simulink model "overtake_QCar"  (R2021a)
settings: Solver=ode1  StartTime=0.0  StopTime=11  FixedStep=1/30  RelTol=1e-3  EnableMultiTasking=on
values from neighbouring files (symbols this model uses):
  animation_update_interval = C*h_fixed    [setup_TP.m]
  enable_CG_trace = 1    [setup_TP.m]
  enable_rearAxle_trace = 1    [setup_TP.m]
  plotAxisLimitMode = 0    [setup_TP.m]
  plotAxisLimits = [-3 4 -3 5]    [setup_TP.m]
  save_anim_frames = 0    [setup_TP.m]
  vehicle_length = 0.256    [setup_TP.m]
  vehicle_width = 0.170    (= 0.17)    [setup_TP.m]
  x0 = [2 6 pi/2]    [setup_TP.m]
undefined symbols (not defined in the file or in its folder): datetime, HIL
libraries: quarc_library x5, simulink x2
settings Model: SimulationMode=external  ExtModeTrigDuration=10000  Creator=Quanser  LastModifiedBy=User
settings SolverCC: AlgebraicLoopSolver=TrustRegion  PositivePriorityOrder=on
settings DataIOCC: ReturnWorkspaceOutputs=off
settings DebuggingCC: PregeneratedLibrarySubsystemCodeDiagnostic=none  SFMachineParentedDataDiag=warning  ArithmeticOperatorsInVariantConditions=warning
settings HardwareCC: ProdBitPerLong=64  ProdLargestAtomicInteger=LongLong  ProdLargestAtomicFloat=Double  ProdLongLongMode=on  ProdHWDeviceType=ARM Compatible->ARM 64-bit (LP64)
settings SFSimCC: CustomCodeUndefinedFunction=UseInterfaceOnly
settings RTWCC: Description=QUARC Linux Nvidia Target (QCar) Using Toolchain  SystemTargetFile=quarc_linux_nvidia.tlc  TemplateMakefile=quarc_default_tmf  Toolchain=QUARC linux_nvidia | gmake (64-bit Windows)  BuildConfiguration=Faster Runs
settings STFCustomTargetCC: TargetLangStandard=C99 (ISO)  ConcurrentExecutionCompliant=on  SystemTargetFile=quarc_linux_nvidia.tlc
settings GRTTargetCC: ParMdlRefBuildCompliant=off  CompOptLevelCompliant=off  CombineOutputUpdateFcns=off  MatFileLogging=off  CPPClassGenCompliant=off  GRTInterface=on  ExtMode=on  ExtModeMexFile=quarc_comm  ExtModeMexArgs='-w -d /tmp -uri %u','tcpip://192.168.2.12:17001'

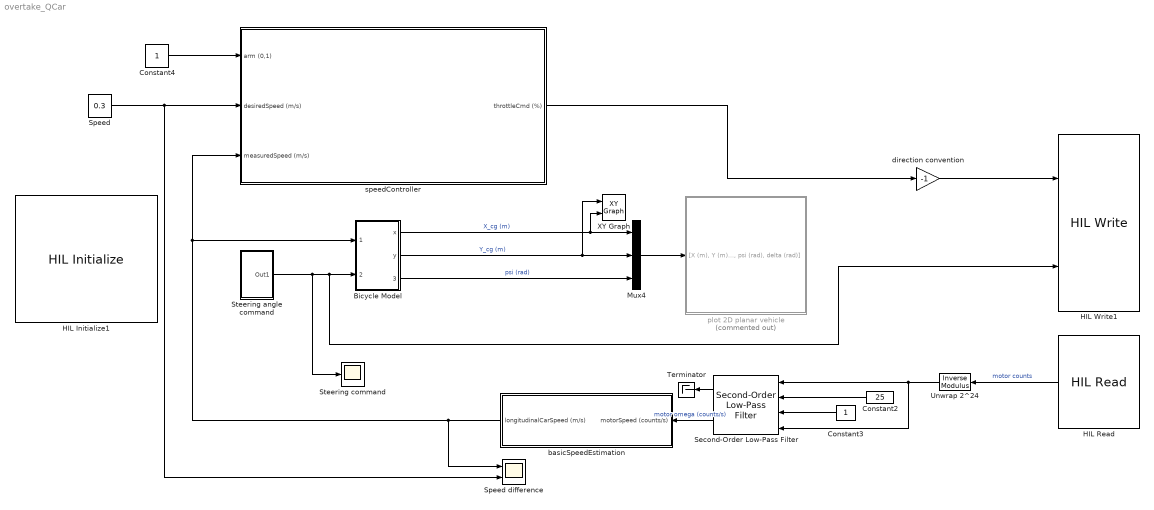
== system overtake_QCar ==
  Bicycle Model : Subsystem
  Constant2 : Constant  Value=25
  Constant3 : Constant
  Constant4 : Constant  VectorParams1D=off
  HIL Initialize1 : quarc_library/Data Acquisition/Generic/Configuration/HIL Initialize  object_name=HIL-1  board_type=qcar  board_number=0  board_options=gyro_fs=125;gyro_rate=47;accel_fs=2;accel_rate=62.5;mag_rate=20;mag_xy=47;mag_z=83;enc1_dir=0;enc2_dir=0;enc3_dir=0;enc4_dir=0;pwm1_dshot=0;pwm2_dshot=0;pwm3_dshot=0;pwm4_dshot=0;pwm5_dshot=0;pwm6_dshot=0;pwm7_dshot=0;steer_bias=0.05;motor_limit=0.3;  exclusive=off  active=on  hardware_clocks=[]  clock_modes=[]  initial_clock_frequencies=[]  set_clock_params_at_start=off  set_clock_params_at_switch_in=off  set_clock_frequencies_at_start=off  set_clock_frequencies_at_switch_in=off  analog_input_channels=[0:6]  analog_input_configurations=[]  analog_input_maximums=[3.3]  analog_input_minimums=[0]  set_analog_input_params_at_start=off  set_analog_input_params_at_switch_in=off  analog_output_channels=[]  analog_output_maximums=[]  analog_output_minimums=[]  initial_analog_outputs=[]  final_analog_outputs=[]  watchdog_analog_outputs=[]  set_analog_output_params_at_start=off  set_analog_output_params_at_switch_in=off  set_analog_outputs_at_start=off  set_analog_outputs_at_switch_in=off  set_analog_outputs_at_terminate=off  set_analog_outputs_at_switch_out=off  set_analog_outputs_on_watchdog=off  digital_input_channels=[24:43]  digital_output_channels=[40]  digital_output_configuration=[]  initial_digital_outputs=[0]  final_digital_outputs=[1]  watchdog_digital_outputs=[]  set_digital_output_params_at_start=off  set_digital_output_params_at_switch_in=off  set_digital_outputs_at_start=on  set_digital_outputs_at_switch_in=off  set_digital_outputs_at_terminate=on  set_digital_outputs_at_switch_out=off  set_digital_outputs_on_watchdog=off  encoder_channels=[0:4]  quadrature=[4 4]  encoder_filter_frequency=100e6/1  initial_encoder_counts=[0]  set_encoder_params_at_start=on  set_encoder_params_at_switch_in=off  set_encoder_counts_at_start=on  set_encoder_counts_at_switch_in=off  pwm_channels=[0:7]  pwm_modes=[0 0]  pwm_frequency=150e6/4096  pwm_configuration=[0]  pwm_alignment=[0]  pwm_polarity=[1]  pwm_leading_deadband=[]  pwm_trailing_deadband=[]  initial_pwm_outputs=[0]  final_pwm_outputs=[0]  watchdog_pwm_outputs=[0]  set_pwm_params_at_start=on  set_pwm_params_at_switch_in=off  set_pwm_outputs_at_start=on  set_pwm_outputs_at_switch_in=off  set_pwm_outputs_at_terminate=on  set_pwm_outputs_at_switch_out=off  set_pwm_outputs_on_watchdog=off  other_output_channels=[1000, 11000:11011]  initial_other_outputs=[0]  final_other_outputs=[0]  watchdog_other_outputs=[]  set_other_outputs_at_start=on  set_other_outputs_at_switch_in=off  set_other_outputs_at_terminate=on  set_other_outputs_at_switch_out=off  set_other_outputs_on_watchdog=off
  HIL Read : quarc_library/Data Acquisition/Generic/Immediate I//O/HIL Read  object_name=HIL-1  analog_channels=[]  encoder_channels=[0]  digital_channels=[]  other_channels=[]  sample_time=qc_get_step_size  active=on  vector_output=off  data_type_mode=Inherit via back propagation  encoder_data_type=double  digital_data_type=boolean
  HIL Write1 : quarc_library/Data Acquisition/Generic/Immediate I//O/HIL Write  object_name=HIL-1  analog_channels=[]  pwm_channels=[0]  digital_channels=[]  other_channels=[1000]  sample_time=-1  active=off  vector_input=off
  Mux4 : Mux  Inputs=3
  Second-Order Low-Pass Filter : quarc_library/Continuous/Second-Order Low-Pass Filter  params_source=External (input ports)  input_width=1  input_zeta=1  input_init=0
  Speed : Constant  Value=0.3
  Speed difference : Scope  NumInputPorts=2
  Steering angle command : Subsystem
  Steering command : Scope
  Terminator : Terminator
  Unwrap 2^24 : quarc_library/Discontinuities/Inverse Modulus  modulus=16777215  output_derivative=off  output_revolutions=off  max_x=Inf  min_x=-Inf
  XY Graph : simulink/Sinks/XY Graph  xmin=-0.5  xmax=0.5  ymin=-1  ymax=4  st=-1
  basicSpeedEstimation : Subsystem
  direction convention : Gain  Gain=-1
  plot 2D planar vehicle : Subsystem  Commented=on  mask(6DoF Animation){axisMode=plotAxisLimitMode, ax=plotAxisLimits, Ts=animation_update_interval, enable_CG_trace=enable_CG_trace, enable_rearAxle_trace=enable_rearAxle_trace, save_anim_frames=save_anim_frames, anim_frame_name_str=char(datetime('now','Format','yyyy-MM-dd_HH_mm_ss')), L=vehicle_length, W=vehicle_width}
      mask prompts: axisMode "Axis Mode (0->auto, 1->fixed, BOTH use Axes Limits below)"; ax "Axes limits [xmin xmax ymin ymax] (m):"; Ts "Time interval between updates (s):"; enable_CG_trace "Enable vehicle CG trace? (0/1)"; enable_rearAxle_trace "Enable rear axle trace? (0/1)"; save_anim_frames "Save animaton frames? (0/1)"; anim_frame_name_str "Animation sequence name (if save frames==1)"; L "Vehicle length (m)"; W "Vehicle width (m)"
      mask help:
      | Create a 2D animated view of a steering vehicle model with tires.
      |
      | Marc Compere
      | CompereM@saic.com
      | created : 22 August 2002
      | modified: 28 Dec 2015
      mask init:
      | Config.axisMode=axisMode;
      | Config.ax=ax;
      | Config.Ts=Ts;
      | Config.enable_CG_trace=enable_CG_trace;
      | Config.enable_rearAxle_trace=enable_rearAxle_trace;
      | Config.save_anim_frames=save_anim_frames;
      | Config.anim_frame_name_str=anim_frame_name_str;
      | Config.L=L;
      | Config.W=W;
      mask Help:
      | <p>This block generates a 3 dimensional display of a simulation trajectory, with the craft orientation displayed during flight</p>
      | 
      | <p>There are two inputs to this block, Position and Euler.  These inputs contain more than one signal as described below.</p>
      | 
      | <p><H4>Block Vector Input - Position</H4>
      | <ul>
      | <li>X Position</li>
      | <li>Y Position</li>
      | <li>Z Position</li>
      | </ul>
      | </p>
      | 
      | <p><H4>Block Vector Input - Euler</H4>
      |     <ul>
      |     <li>Roll Attitude</li>
      |     <li>Pitch Attitude</li>
      |     <li>Yaw Attitude</li>
      |    </ul>
      |    </p>
  speedController : Subsystem
  wires:
  Unwrap 2^24/1 -> Second-Order Low-Pass Filter/1, Second-Order Low-Pass Filter/4
  HIL Read/1 -> Unwrap 2^24/1  "motor counts"
  speedController/1(throttleCmd (%)) -> direction convention/1
  Constant3/1 -> Second-Order Low-Pass Filter/3
  basicSpeedEstimation/1(longitudinalCarSpeed (m/s)) -> Speed difference/1, speedController/3(measuredSpeed (m/s)), Bicycle Model/1(velocity)
  Speed/1 -> Speed difference/2, speedController/2(desiredSpeed (m/s))
  Mux4/1 -> plot 2D planar vehicle/1("[X (m), Y (m), psi (rad), delta (rad)]")
  Constant2/1 -> Second-Order Low-Pass Filter/2
  Second-Order Low-Pass Filter/2 -> basicSpeedEstimation/1(motorSpeed (counts/s))  "motor omega (counts/s)"
  direction convention/1 -> HIL Write1/1
  Constant4/1 -> speedController/1(arm (0,1))
  Bicycle Model/1(x) -> XY Graph/2, Mux4/1  "X_cg (m)"
  Bicycle Model/2(y) -> XY Graph/1, Mux4/2  "Y_cg (m)"
  Bicycle Model/3(theta) -> Mux4/3  "psi (rad)"
  Steering angle command/1(Out1) -> Steering command/1, HIL Write1/2, Bicycle Model/2(gamma)
  Second-Order Low-Pass Filter/1 -> Terminator/1

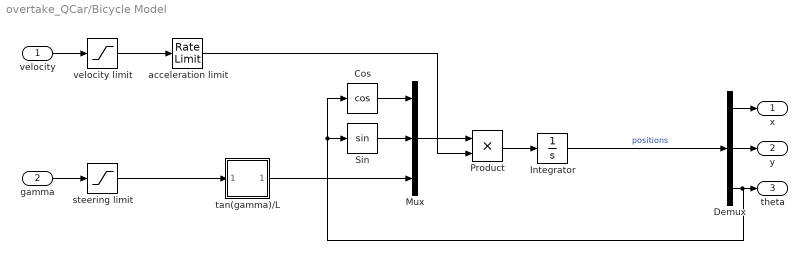
== system overtake_QCar/Bicycle Model ==
  velocity : Inport
  gamma : Inport  Port=2
  Cos : Trigonometry  Operator=cos
  Demux : Demux  Outputs=3
  Integrator : Integrator  InitialCondition=x0
  Mux : Mux  Inputs=3
  Product : Product
  Sin : Trigonometry
  acceleration limit : RateLimiter  RisingSlewLimit=2  FallingSlewLimit=-2  SampleTimeMode=inherited
  steering limit : Saturate  UpperLimit=1  LowerLimit=-1
  tan(gamma)/L : Subsystem
  velocity limit : Saturate  UpperLimit=5  LowerLimit=-5
  x : Outport
  y : Outport  Port=2
  theta : Outport  Port=3
  wires:
  velocity/1 -> velocity limit/1
  velocity limit/1 -> acceleration limit/1
  gamma/1 -> steering limit/1
  steering limit/1 -> tan(gamma)/L/1(In1)
  tan(gamma)/L/1(Out1) -> Mux/3
  Mux/1 -> Product/1
  acceleration limit/1 -> Product/2
  Product/1 -> Integrator/1
  Integrator/1 -> Demux/1  "positions"
  Demux/3 -> Cos/1, Sin/1, theta/1
  Demux/1 -> x/1
  Demux/2 -> y/1
  Cos/1 -> Mux/1
  Sin/1 -> Mux/2

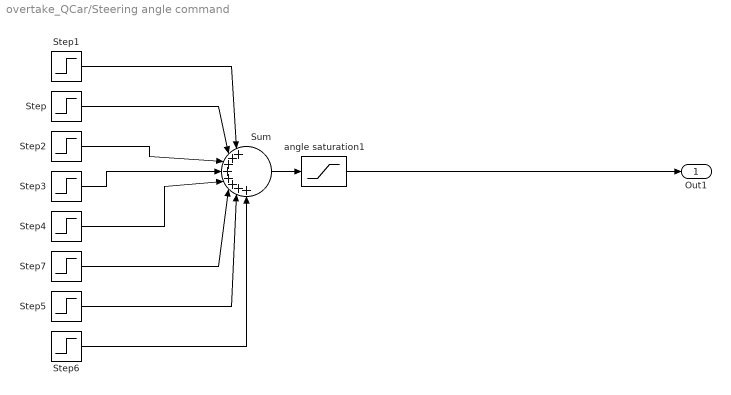
== system overtake_QCar/Steering angle command ==
  Step : Step  Time=3  After=0.37
  Step1 : Step  Time=2  After=-0.37
  Step2 : Step  Time=4.5  After=0.37
  Step3 : Step  Time=5.5  After=-0.37
  Step4 : Step  Time=6.5  After=0.37
  Step5 : Step  Time=9.1  After=-0.37
  Step6 : Step  Time=10.2  After=0.37
  Step7 : Step  Time=7.5  After=-0.37
  Sum : Sum  Inputs=|++++++++
  angle saturation1 : Saturate
  Out1 : Outport
  wires:
  Step/1 -> Sum/2
  Step3/1 -> Sum/4
  Step7/1 -> Sum/6
  Step2/1 -> Sum/3
  Step5/1 -> Sum/7
  Step1/1 -> Sum/1
  Step4/1 -> Sum/5
  Sum/1 -> angle saturation1/1
  Step6/1 -> Sum/8
  angle saturation1/1 -> Out1/1

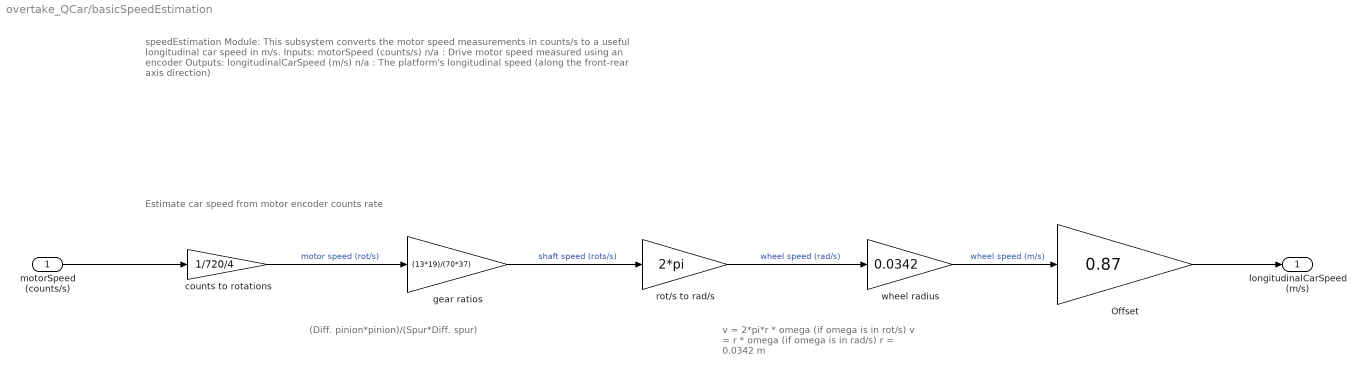
== system overtake_QCar/basicSpeedEstimation ==
  note: Estimate car speed from motor encoder counts rate
  note: v = 2*pi*r * omega (if omega is in rot/s)
      | v = r * omega (if omega is in rad/s)
      | r = 0.0342 m
  note: (Diff. pinion*pinion)/(Spur*Diff. spur)
  note: speedEstimation Module:
      |
      | This subsystem converts the motor speed measurements in counts/s to a useful longitudinal car speed in m/s.
      |
      | Inputs:
      | motorSpeed (counts/s) n/a : Drive motor speed measured using an encoder
      |
      | Outputs:
      | longitudinalCarSpeed (m/s) n/a : The platform's longitudinal speed (along the front-rear axis direction)
  motorSpeed (counts/s) : Inport
  Offset : Gain  Gain=0.87
  counts to rotations : Gain  Gain=1/720/4
  gear ratios : Gain  Gain=(13*19)/(70*37)
  rot/s to rad/s : Gain  Gain=2*pi
  wheel radius : Gain  Gain=0.0342
  longitudinalCarSpeed (m/s) : Outport  VectorParamsAs1DForOutWhenUnconnected=off
  wires:
  motorSpeed (counts/s)/1 -> counts to rotations/1
  rot/s to rad/s/1 -> wheel radius/1  "wheel speed (rad/s)"
  counts to rotations/1 -> gear ratios/1  "motor speed (rot/s)"
  wheel radius/1 -> Offset/1  "wheel speed (m/s)"
  gear ratios/1 -> rot/s to rad/s/1  "shaft speed (rots/s)"
  Offset/1 -> longitudinalCarSpeed (m/s)/1

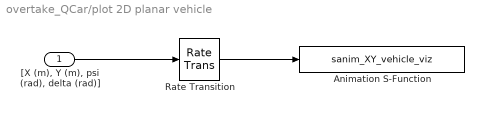
== system overtake_QCar/plot 2D planar vehicle ==
  "[X (m), Y (m), psi (rad), delta (rad)]" : Inport
  Animation S-Function : S-Function  FunctionName=sanim_XY_vehicle_viz  Parameters=Config  SFunctionDeploymentMode=off  EnableBusSupport=off
  Rate Transition : RateTransition  Integrity=off
  wires:
  "[X (m), Y (m), psi (rad), delta (rad)]"/1 -> Rate Transition/1
  Rate Transition/1 -> Animation S-Function/1

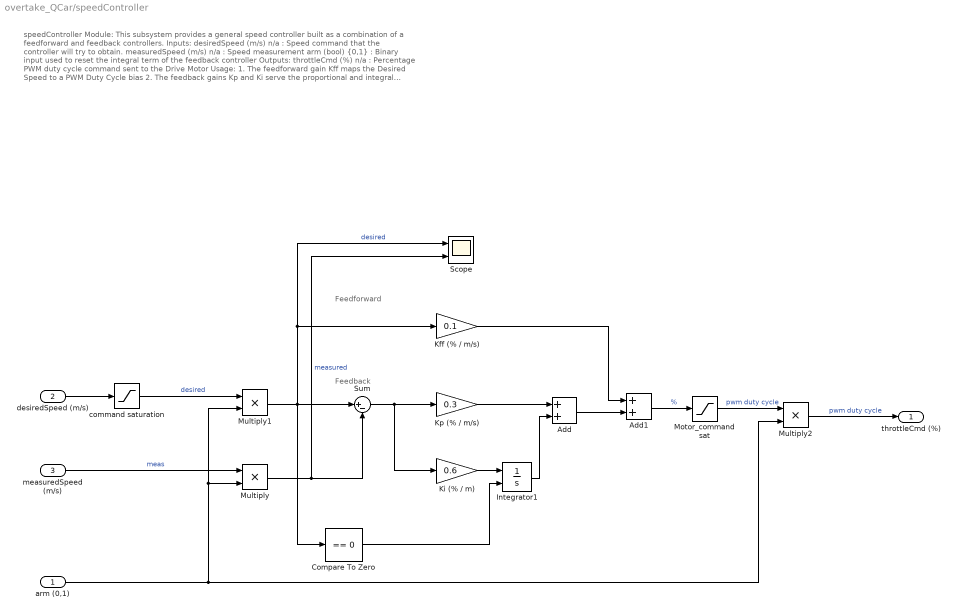
== system overtake_QCar/speedController ==
  note: speedController Module:
      |
      | This subsystem provides a general speed controller built as a combination of a feedforward and feedback controllers.
      |
      | Inputs:
      | desiredSpeed (m/s) n/a : Speed command that the controller will try to obtain.
      | measuredSpeed (m/s) n/a : Speed measurement
      | arm (bool) {0,1} : Binary input used to reset the integral term of the feedback controller
      |
      | Outputs:
      | throttleCmd (%) n/a : Percentage PWM duty cycle command sent to the Drive Motor
      |
      | Usage:
      | 1. The feedforward gain Kff maps the Desired Speed to a PWM Duty Cycle bias
      | 2. The feedback gains Kp and Ki serve the proportional and integral terms to output corrections to the PWM Duty Cycle so as to regulate the desired speed.
  note: Feedback
  note: Feedforward
  arm (0,1) : Inport
  desiredSpeed (m/s) : Inport  Port=2
  measuredSpeed (m/s) : Inport  Port=3
  Add : Sum
  Add1 : Sum
  Compare To Zero : simulink/Logic and Bit Operations/Compare To Zero  relop===  OutDataTypeStr=boolean
  Integrator1 : Integrator  ExternalReset=either  LimitOutput=on  UpperSaturationLimit=0.1  LowerSaturationLimit=-0.1
  Kff (% / m/s) : Gain  Gain=0.1
  "Ki (% / m) " : Gain  Gain=0.6
  Kp (% / m/s) : Gain  Gain=0.3
  Motor_command sat : Saturate  LinearizeAsGain=off
  Multiply : Product
  Multiply1 : Product
  Multiply2 : Product
  Scope : Scope  NumInputPorts=2
  Sum : Sum  Inputs=|+-
  command saturation : Saturate
  throttleCmd (%) : Outport  VectorParamsAs1DForOutWhenUnconnected=off
  wires:
  desiredSpeed (m/s)/1 -> command saturation/1
  "Ki (% / m) "/1 -> Integrator1/1
  Sum/1 -> Kp (% / m/s)/1, "Ki (% / m) "/1
  Kff (% / m/s)/1 -> Add1/1
  Compare To Zero/1 -> Integrator1/2
  Kp (% / m/s)/1 -> Add/1
  Multiply2/1 -> throttleCmd (%)/1  "pwm duty cycle"
  Integrator1/1 -> Add/2
  Multiply1/1 -> Scope/1, Kff (% / m/s)/1, Sum/1, Compare To Zero/1  "desired"
  Add1/1 -> Motor_command sat/1  "%"
  Motor_command sat/1 -> Multiply2/1  "pwm duty cycle"
  Add/1 -> Add1/2
  Multiply/1 -> Scope/2, Sum/2  "measured"
  measuredSpeed (m/s)/1 -> Multiply/1  "meas"
  arm (0,1)/1 -> Multiply2/2, Multiply/2, Multiply1/2
  command saturation/1 -> Multiply1/1  "desired"

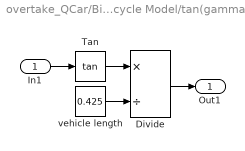
== system overtake_QCar/Bicycle Model/tan(gamma)//L ==
  In1 : Inport
  Divide : Product  Inputs=*/
  Tan : Trigonometry  Operator=tan
  vehicle length : Constant  Value=0.425
  Out1 : Outport
  wires:
  Tan/1 -> Divide/1
  vehicle length/1 -> Divide/2
  In1/1 -> Tan/1
  Divide/1 -> Out1/1
